simulink model "diagramme"  (R2022b)
settings: Solver=VariableStepAuto  StartTime=0.0  StopTime=10.0  RelTol=1e-3
settings Model: Creator=taha  LastModifiedBy=taha

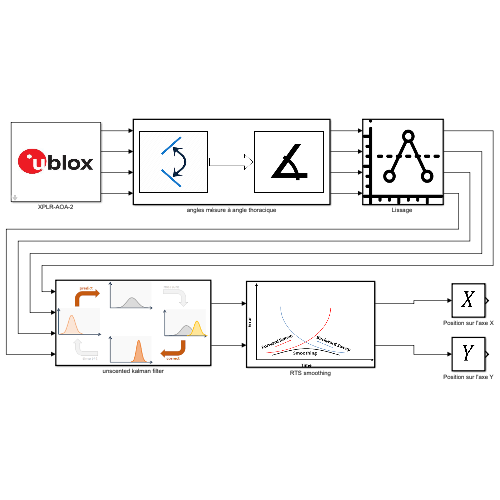
[thumbnail: Simulink's stored preview of the top-level diagram]
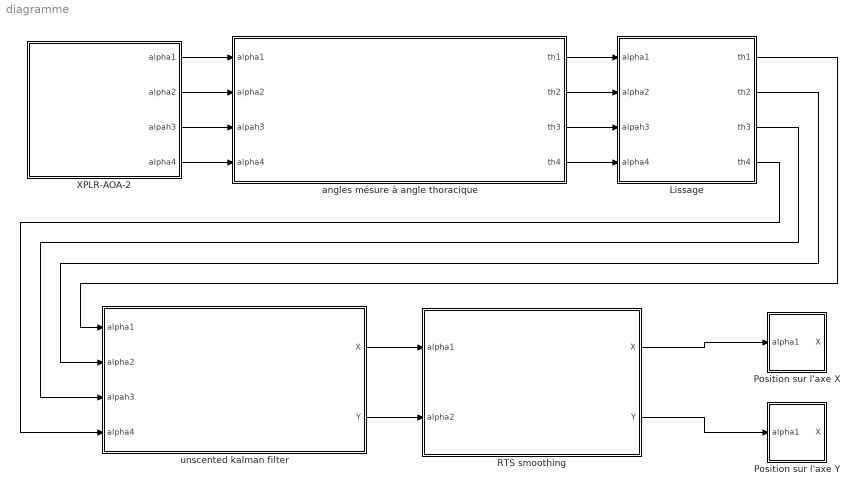
== system diagramme ==
  "Lissage " : MATLAB Function  TreatAsAtomicUnit=on
  Position sur l'axe X : MATLAB Function  TreatAsAtomicUnit=on
  Position sur l'axe Y : MATLAB Function  TreatAsAtomicUnit=on
  RTS smoothing : MATLAB Function  TreatAsAtomicUnit=on
  XPLR-AOA-2 : Subsystem
      mask DialogControl Control1 Prompt: (Add text here)
      mask Display: image('C:\Users\taha\Desktop\stage PFE\Kalman Filter\EKF matlab\Ublox XPLR-AOA-2\image\Ublox.jpg');
  angles mésure à angle thoracique : MATLAB Function  TreatAsAtomicUnit=on
  unscented kalman filter : MATLAB Function  TreatAsAtomicUnit=on
  wires:
  XPLR-AOA-2/1(alpha1) -> angles mésure à angle thoracique/1(alpha1)
  XPLR-AOA-2/2(alpha2) -> angles mésure à angle thoracique/2(alpha2)
  XPLR-AOA-2/3(alpah3) -> angles mésure à angle thoracique/3(alpah3)
  XPLR-AOA-2/4(alpha4) -> angles mésure à angle thoracique/4(alpha4)
  angles mésure à angle thoracique/1(th1) -> "Lissage "/1(alpha1)
  angles mésure à angle thoracique/2(th2) -> "Lissage "/2(alpha2)
  angles mésure à angle thoracique/3(th3) -> "Lissage "/3(alpah3)
  angles mésure à angle thoracique/4(th4) -> "Lissage "/4(alpha4)
  "Lissage "/2(th2) -> unscented kalman filter/2(alpha2)
  "Lissage "/1(th1) -> unscented kalman filter/1(alpha1)
  "Lissage "/3(th3) -> unscented kalman filter/3(alpah3)
  "Lissage "/4(th4) -> unscented kalman filter/4(alpha4)
  unscented kalman filter/1(X) -> RTS smoothing/1(alpha1)
  unscented kalman filter/2(Y) -> RTS smoothing/2(alpha2)
  RTS smoothing/1(X) -> Position sur l'axe X/1(alpha1)
  RTS smoothing/2(Y) -> Position sur l'axe Y/1(alpha1)

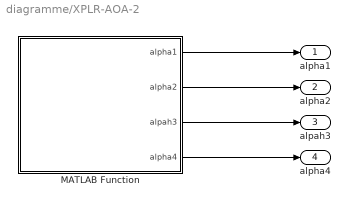
== system diagramme/XPLR-AOA-2 ==
  MATLAB Function : MATLAB Function  TreatAsAtomicUnit=on
  alpha1 : Outport
  alpha2 : Outport  Port=2
  alpah3 : Outport  Port=3
  alpha4 : Outport  Port=4
  wires:
  MATLAB Function/2(alpha2) -> alpha2/1
  MATLAB Function/3(alpah3) -> alpah3/1
  MATLAB Function/4(alpha4) -> alpha4/1
  MATLAB Function/1(alpha1) -> alpha1/1

== matlab function diagramme/angles mésure à angle thoracique ==
  data: th1 output; th2 output; th3 output; th4 output; alpha1 input; alpha2 input; alpah3 input; alpha4 input
function [th1,th2,th3,th4] = fun(alpha1,alpha2,alpah3,alpha4)

== matlab function diagramme/XPLR-AOA-2/MATLAB Function ==
  data: alpha1 output; alpha2 output; alpah3 output; alpha4 output
function [alpha1,alpha2,alpah3,alpha4] = fun()

== matlab function diagramme/Lissage  ==
  data: th1 output; th2 output; th3 output; th4 output; alpha1 input; alpha2 input; alpah3 input; alpha4 input
function [th1,th2,th3,th4] = fun(alpha1,alpha2,alpah3,alpha4)

== matlab function diagramme/unscented kalman filter ==
  data: X output; Y output; alpha1 input; alpha2 input; alpah3 input; alpha4 input
function [X,Y] = fun(alpha1,alpha2,alpah3,alpha4)

== matlab function diagramme/RTS smoothing ==
  data: X output; Y output; alpha1 input; alpha2 input
function [X,Y] = fun(alpha1,alpha2)

== matlab function diagramme/Position sur l'axe X ==
  data: X output; alpha1 input
function X  = fun(alpha1)

== matlab function diagramme/Position sur l'axe Y ==
  data: X output; alpha1 input
function X  = fun(alpha1)
